simulink model "manipulator_cl"  (R2018b)
settings: Solver=ode45  StartTime=0.0  StopTime=4  RelTol=1e-9
values from neighbouring files (symbols this model uses):
  alpha_rel = 60*pi/180    (= 1.0471975512)    [comparison_phtitop.m]
  kp1 = 160    [comparison_phtitop.m]    (also in manipulator_phpfem.m)
  kp2 = 60    [comparison_phtitop.m]    (also in manipulator_phpfem.m)
  kv1 = 11    [comparison_phtitop.m]    (also in manipulator_phpfem.m)
  Kv2 = 1.1    [comparison_phtitop.m]
  rad_deg = 180/pi    (= 57.2957795131)    [comparison_phtitop.m]
  sys_phode = ss(J_ode * Q_ode, B_ode, B_ode'* Q_ode, 0)    [manipulator_phpfem.m]
  sys_titop = directDynamicsSuper*tf(1, [1, 0])    [manipulatorAlvaro_titop.m]    (also in manipulatorSanfe_titop.m)
settings Model: Creator=a.brugnoli  LastModifiedBy=a.brugnoli

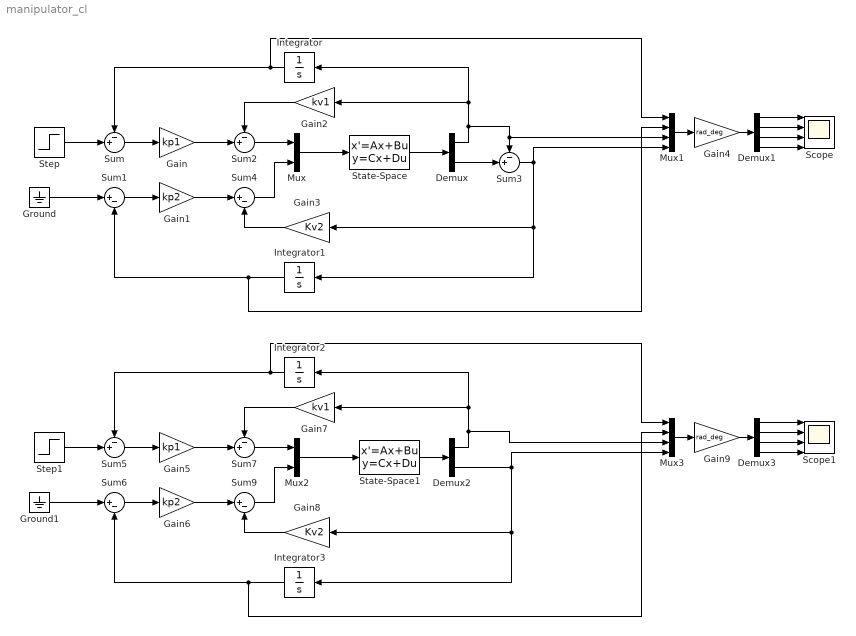
== system manipulator_cl ==
  Demux : Demux  Outputs=2
  Demux1 : Demux
  Demux2 : Demux  Outputs=2
  Demux3 : Demux
  Gain : Gain  Gain=kp1
  Gain1 : Gain  Gain=kp2
  Gain2 : Gain  Gain=kv1
  Gain3 : Gain  Gain=Kv2
  Gain4 : Gain  Gain=rad_deg
  Gain5 : Gain  Gain=kp1
  Gain6 : Gain  Gain=kp2
  Gain7 : Gain  Gain=kv1
  Gain8 : Gain  Gain=Kv2
  Gain9 : Gain  Gain=rad_deg
  Ground : Ground
  Ground1 : Ground
  Integrator{,1..3} (4 alike) : Integrator
  Mux : Mux  Inputs=2
  Mux1 : Mux
  Mux2 : Mux  Inputs=2
  Mux3 : Mux
  Scope : Scope  NumInputPorts=4
  Scope1 : Scope  NumInputPorts=4
  State-Space : StateSpace  A=sys_phode.A  B=sys_phode.B  C=sys_phode.C  D=sys_phode.D  InitialCondition=0
  State-Space1 : StateSpace  A=sys_titop.A  B=sys_titop.B  C=sys_titop.C  D=sys_titop.D  InitialCondition=0
  Step : Step  After=alpha_rel  SampleTime=0
  Step1 : Step  After=alpha_rel  SampleTime=0
  Sum{,2..3,5,7} (5 alike) : Sum  Inputs=-+|
  Sum{1,4,6,9} (4 alike) : Sum  Inputs=|+-
  wires:
  State-Space/1 -> Demux/1
  Demux/1 -> Mux1/3, Sum3/1, Gain2/1, Integrator/1
  Ground/1 -> Sum1/1
  Integrator/1 -> Mux1/1, Sum/1
  Sum3/1 -> Mux1/4, Gain3/1, Integrator1/1
  Sum/1 -> Gain/1
  Mux/1 -> State-Space/1
  Integrator1/1 -> Mux1/2, Sum1/2
  Gain/1 -> Sum2/2
  Sum2/1 -> Mux/1
  Gain2/1 -> Sum2/1
  Demux/2 -> Sum3/2
  Sum1/1 -> Gain1/1
  Gain3/1 -> Sum4/2
  Gain1/1 -> Sum4/1
  Sum4/1 -> Mux/2
  Step/1 -> Sum/2
  Mux1/1 -> Gain4/1
  Demux1/3 -> Scope/3
  Demux1/4 -> Scope/4
  Gain4/1 -> Demux1/1
  Demux1/2 -> Scope/2
  Demux1/1 -> Scope/1
  Step1/1 -> Sum5/2
  Gain5/1 -> Sum7/2
  Integrator2/1 -> Mux3/1, Sum5/1
  Gain9/1 -> Demux3/1
  Demux3/4 -> Scope1/4
  Demux3/2 -> Scope1/2
  Gain8/1 -> Sum9/2
  Sum5/1 -> Gain5/1
  Demux3/3 -> Scope1/3
  State-Space1/1 -> Demux2/1
  Demux3/1 -> Scope1/1
  Sum6/1 -> Gain6/1
  Mux2/1 -> State-Space1/1
  Sum7/1 -> Mux2/1
  Gain6/1 -> Sum9/1
  Integrator3/1 -> Mux3/2, Sum6/2
  Demux2/1 -> Mux3/3, Gain7/1, Integrator2/1
  Ground1/1 -> Sum6/1
  Demux2/2 -> Integrator3/1, Gain8/1, Mux3/4
  Sum9/1 -> Mux2/2
  Mux3/1 -> Gain9/1
  Gain7/1 -> Sum7/1
